simulink model "ALL_JP360_DBW_V6_5_1103"  (R2022a)
settings: Solver=FixedStepAuto  StartTime=0.0  StopTime=inf  FixedStep=0.01  RelTol=1e-3  EnableMultiTasking=on
model workspace (MAT data in the model file):
  g = 9.8
undefined symbols (not defined in the file or in its folder): canChannel, delta_v_p, IPM_Line_C0, IPM_Line_C1, IPM_Line_C2, IPM_Line_C3, M, M_p, MRR_ObjDistX, MRR_ObjDistY, MRR_ObjFusionCamID, MRR_ObjFusionSig, MRR_ObjID, MRR_ObjRelVelX, MRR_ObjRelVelY, MRR_ObjType, MRR_ObjUpdFlg, none, obj_vaild, untracktime, V, videoinput
libraries: canfdmsglib x230, canfdlib x76, slpidlib x24, simulink x18, dspstat3 x14, ctrlSharedLib x1, simulink_extras x1, imaqlib x1, realtime_pacer_lib x1, dspvision x1, visionsinks x1
(part 1 of 55)
settings Model: Creator=35528  LastModifiedBy=91388
settings SolverCC: PositivePriorityOrder=on  AutoInsertRateTranBlk=on
settings OptimizationCC: DefaultParameterBehavior=Inlined  GainParamInheritBuiltInType=on  UseFloatMulNetSlope=on  DefaultUnderspecifiedDataType=single  UseSpecifiedMinMax=on  InlineInvariantSignals=on  EnhancedBackFolding=on  CachingGlobalReferences=on  BitwiseOrLogicalOp=Bitwise operator  PassReuseOutputArgsAs=Individual arguments  ZeroExternalMemoryAtStartup=off  ZeroInternalMemoryAtStartup=off  NoFixptDivByZeroProtection=on  EfficientFloat2IntCast=on  OptimizeBlockOrder=speed  DifferentSizesBufferReuse=on  MultiThreadedLoops=on  EfficientTunableParamExpr=on
settings DebuggingCC: ParameterOverflowMsg=none  ParameterTunabilityLossMsg=error
settings ModelReferenceCC: ModelReferenceMinAlgLoopOccurrences=on
settings SFSimCC: MATLABDynamicMemAlloc=off
settings RTWCC: SystemTargetFile=ert.tlc  GenCodeOnly=on  PackageGeneratedCodeAndArtifacts=on  TemplateMakefile=ert_default_tmf  RetainRTWFile=on  BuildConfiguration=Faster Runs  CheckMdlBeforeBuild=Warning
settings CodeAppCC: ForceParamTrailComments=on  IgnoreCustomStorageClasses=off  OperatorAnnotations=on  SimulinkDataObjDesc=on  SFDataObjDesc=on  MATLABFcnDesc=on  InsertBlockDesc=on  StateflowObjectComments=on  MATLABSourceComments=on  ReqsInCode=on
settings ERTTargetCC: TargetLangStandard=C99 (ISO)  GenerateSampleERTMain=on  SuppressErrorStatus=on  SupportNonFinite=off  InlinedParameterPlacement=NonHierarchical  MultiInstanceErrorCode=Warning  RootIOFormat=Part of model data structure  ERTCustomFileTemplate=example_file_process.tlc

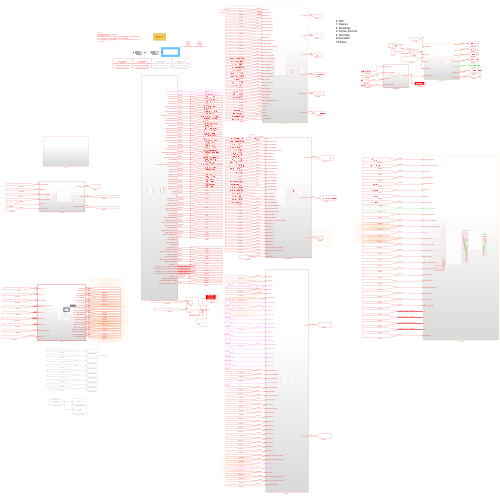
[thumbnail: Simulink's stored preview of the top-level diagram]
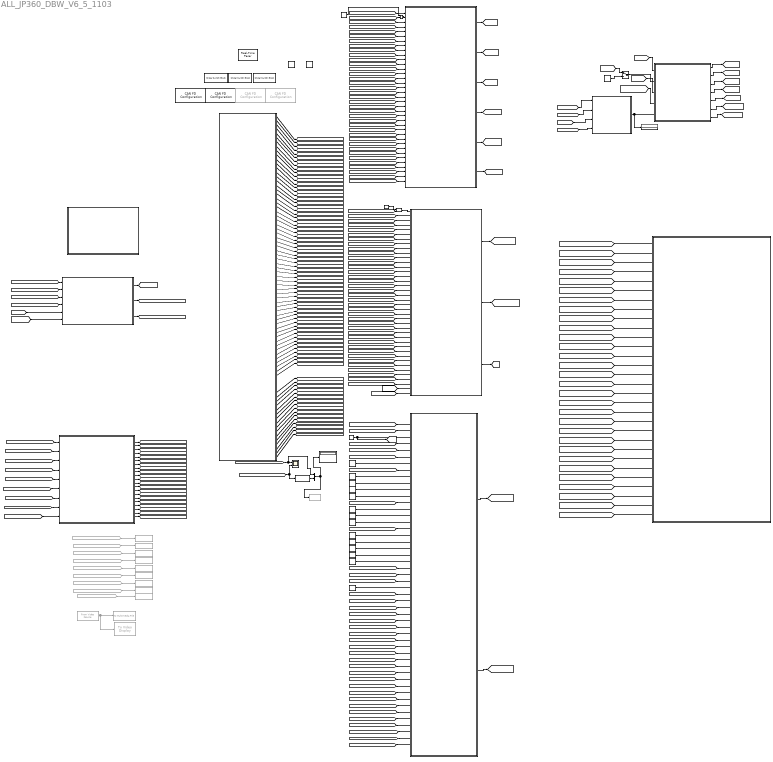
== system ALL_JP360_DBW_V6_5_1103 ==
  note: 0: OFF
      | 1: Passive
      | 2: Stand-By
      | 3: Active-Control
      | 5: Override
      | 6: Standstill
      | 7: Failure
  note: 注意事项
      | 1.添加Real-Time Pacer文件夹到路径下
      | 2.双击20230916.mat文件
      | 3.连接CANoe硬件（每次打开模型前最好电脑连接CANoe硬件，否则CAN配置会变），channel3对应公CAN，channel4对应1V1R私有CAN
      | 4.如果发现CAN配置变为了MathWork...，那么运行ALL_JP360_DBW_V2_2m.m文件，运行两次！！！！！！！！！
  ACC : Constant  OutDataTypeStr=boolean
  ACC_Control : Subsystem
  CAN FD Configuration1 : canfdlib/CAN FD Configuration  Device=Vector VN1640A 1 (Channel 3)  DeviceMenu=Vector VN1640A 1 (Channel 3)  BusFrequency=20  ObjConstructor=canChannel('Vector', 'VN1640A 1', 3, 'ProtocolMode', 'CAN FD')  ArbitrationBusSpeed=500000  ArbitrationPrescaler=5  ArbitrationSJW=8  ArbitrationTSEG1=31  ArbitrationTSEG2=8  DataBusSpeed=2000000  DataPrescaler=2  DataSJW=2  DataTSEG1=7  DataTSEG2=2  AckMode=Normal  BlockHandle=69358.0004
      settings: SourceProductBaseCode=VN
  CAN FD Configuration2 : canfdlib/CAN FD Configuration  Device=Vector VN1640A 1 (Channel 4)  DeviceMenu=Vector VN1640A 1 (Channel 4)  BusFrequency=20  ObjConstructor=canChannel('Vector', 'VN1640A 1', 4, 'ProtocolMode', 'CAN FD')  ArbitrationBusSpeed=500000  ArbitrationPrescaler=5  ArbitrationSJW=8  ArbitrationTSEG1=31  ArbitrationTSEG2=8  DataBusSpeed=2000000  DataPrescaler=2  DataSJW=2  DataTSEG1=7  DataTSEG2=2  AckMode=Normal  BlockHandle=69359.0004
      settings: SourceProductBaseCode=VN
  CAN FD Configuration3 : canfdlib/CAN FD Configuration  Commented=on  Device=MathWorks Virtual 1 (Channel 1)  DeviceMenu=MathWorks Virtual 1 (Channel 1)  BusFrequency=20  ObjConstructor=canChannel('MathWorks', 'Virtual 1', 1, 'ProtocolMode', 'CAN FD')  ArbitrationBusSpeed=1000000  ArbitrationPrescaler=5  ArbitrationSJW=8  ArbitrationTSEG1=31  ArbitrationTSEG2=8  DataBusSpeed=8000000  DataPrescaler=2  DataSJW=2  DataTSEG1=7  DataTSEG2=2  AckMode=Normal  BlockHandle=69360.0004
      settings: SourceProductBaseCode=VN
  CAN FD Configuration4 : canfdlib/CAN FD Configuration  Commented=on  Device=MathWorks Virtual 1 (Channel 1)  DeviceMenu=MathWorks Virtual 1 (Channel 1)  BusFrequency=20  ObjConstructor=canChannel('MathWorks', 'Virtual 1', 1, 'ProtocolMode', 'CAN FD')  ArbitrationBusSpeed=1000000  ArbitrationPrescaler=5  ArbitrationSJW=8  ArbitrationTSEG1=31  ArbitrationTSEG2=8  DataBusSpeed=8000000  DataPrescaler=2  DataSJW=2  DataTSEG1=7  DataTSEG2=2  AckMode=Normal  BlockHandle=69361.0004
      settings: SourceProductBaseCode=VN
  CIPV1 : Subsystem  TreatAsAtomicUnit=on
  CanbusControl : Subsystem
  Constant{10,44,47..48} (4 alike) : Constant  Value=150  OutDataTypeStr=single
  Constant{11,15,21,32} (4 alike) : Constant  Value=100  OutDataTypeStr=single
  Constant{12,19,22,33} (4 alike) : Constant  Value=20  OutDataTypeStr=single
  Constant40 : Constant  Value=0  OutDataTypeStr=int8
  Constant43 : Constant  Value=0  OutDataTypeStr=single
  Constant7 : Constant  OutDataTypeStr=single
  DCLC : Constant  OutDataTypeStr=boolean
  DCLC1 : Subsystem
  Data Store Memory : DataStoreMemory  DataStoreName=acc_change_mode  ReadBeforeWriteMsg=warning  WriteAfterWriteMsg=warning  WriteAfterReadMsg=warning  ShowAdditionalParam=off
  Data Store Memory1 : DataStoreMemory  DataStoreName=SpdSetValue  ReadBeforeWriteMsg=warning  WriteAfterWriteMsg=warning  WriteAfterReadMsg=warning  ShowAdditionalParam=off
  Data Type Conversion : DataTypeConversion  OutDataTypeStr=single  SaturateOnIntegerOverflow=off  RndMeth=Floor
  Display : Display
  Display1 : Display
  Error : Subsystem
  From Video Device : imaqlib/From Video Device  Commented=on  DeviceMenu=(none)  Device=winvideo 2 (SY 1080P camera)  ObjConstructor=videoinput('winvideo', 2)  VideoFormatMenu=(none)  VideoFormat=YUY2_352x288  VideoSource=input1  ROIPosition=[0 0 288 352]  EnableHWTrigger=off  TriggerConfiguration=none/none  SampleTime=0.03  OutputPortsMode=One multidimensional signal  DataType=single  CanDoHWTrigger=no  ReturnedColorSpace=rgb  BlockHandle=66699.0001  ROIWidth=352  ROIHeight=288  ROIColumn=0  ROIRow=0  EngXMLPath=D:\Program Files\MATLAB\R2022a\toolbox\imaq\imaq\private  DevXMLPath=C:\ProgramData\MATLAB\SupportPackages\R2022a\toolbox\imaq\supportpackages\genericvideo\adaptor\win64  EngLibPath=D:\Program Files\MATLAB\R2022a\toolbox\imaq\imaqblks\imaqmex\win64  ColorSpace=rgb  BayerSensorAlignment=grbg  ImaqMode=off
  From109 : From  Commented=on  GotoTag=MRR_obj_1_32
  From113 : From  Commented=on  GotoTag=ABS_VehSpdLgt
  From161 : From  Commented=on  GotoTag=ESP_YawRate
  From162 : From  Commented=on  GotoTag=VR_ADCU_IPM_Line_01_0x640FromOutData
  From163 : From  Commented=on  GotoTag=VR_ADCU_IPM_Line_02_0x641FromOutData
  From164 : From  Commented=on  GotoTag=VR_ADCU_IPM_Line_03_0x642FromOutData
  From165 : From  Commented=on  GotoTag=VR_ADCU_IPM_Line_04_0x643FromOutData
  From166 : From  Commented=on  GotoTag=SAS_SteerWheelAngle
  From167 : From  Commented=on  GotoTag=IPM_obj_1_20
  LKA : Constant  OutDataTypeStr=boolean
  LKA_Control : Subsystem
  Manual Switch : ManualSwitch
  MsgFromCAN : Subsystem
  MsgToCAN : Subsystem
  Mux : Mux  Inputs=2
  Product : Product
  Product1 : Product
  Real-Time Pacer : realtime_pacer_lib/Real-Time Pacer  simTimePerRealTime=1
      settings: SourceProductName=Real-Time Pacer
  Scope : Scope  NumInputPorts=2
  Slider Switch : SliderSwitchBlock
      settings: Values={{'Off', 'On'}, [0 1]}
  Slider Switch1 : SliderSwitchBlock
      settings: Values={{'Off', 'On'}, [0 1]}
  Slider Switch2 : SliderSwitchBlock
      settings: Values={{'Off', 'On'}, [0 1]}
  Subsystem1 : Subsystem
  To File : ToFile  Commented=on  Filename=EMS_HMI110_2.mat  SaveFormat=Timeseries
  To Multimedia File : dspvision/To Multimedia File  Commented=on  outputFilename=output.avi  streamSelection=Video only  videoCompressor=None (uncompressed)  audioCompressor=None (uncompressed)  imagePorts=One multidimensional signal  fileType=AVI  audioDatatype=16-bit integer  fourcc=RGB  videoQuality=75  mj2000CompFactor=10
  To Video Display : visionsinks/To Video Display  Commented=on  windowSizeMode=Normal  openAtMdlStart=on  fullScreen=off  videoWindowX=536805376  videoWindowY=536805376  saveWindowSize=off  videoWindowWidth=1280  videoWindowHeight=720  inputColorFormat=RGB  inputType=Obsolete  imagePorts=One multidimensional signal  OutputDevice=On-screen video monitor  dataOrg=Column-major  isWindowOpen=off
  To Workspace1 : ToWorkspace  Commented=on  VariableName=MRR_obj_1_32  SaveFormat=Timeseries  SampleTime=-1
  To Workspace2 : ToWorkspace  Commented=on  VariableName=ABS_VehSpdLgt  SaveFormat=Timeseries  SampleTime=-1
  To Workspace3 : ToWorkspace  Commented=on  VariableName=ESP_YawRate  SaveFormat=Timeseries  SampleTime=-1
  To Workspace4 : ToWorkspace  Commented=on  VariableName=VR_ADCU_IPM_Line_01_0x640FromOutData  SaveFormat=Timeseries  SampleTime=-1
  To Workspace5 : ToWorkspace  Commented=on  VariableName=VR_ADCU_IPM_Line_02_0x641FromOutData  SaveFormat=Timeseries  SampleTime=-1
  To Workspace6 : ToWorkspace  Commented=on  VariableName=VR_ADCU_IPM_Line_03_0x642FromOutData  SaveFormat=Timeseries  SampleTime=-1
  To Workspace7 : ToWorkspace  Commented=on  VariableName=VR_ADCU_IPM_Line_04_0x643FromOutData  SaveFormat=Timeseries  SampleTime=-1
  To Workspace8 : ToWorkspace  Commented=on  VariableName=SAS_SteerWheelAngle  SaveFormat=Timeseries  SampleTime=-1
  To Workspace9 : ToWorkspace  Commented=on  VariableName=IPM_obj_1_20  SaveFormat=Timeseries  SampleTime=-1
  button : Subsystem
  wires:
  [IPM_obj_1_20] -> CIPV1/9(IPM_obj_1_20)
  MsgFromCAN/43(Output8) -> [ESP_Algt]
  [EMS_IndicatedEngError] -> ACC_Control/16(EMS_IndicatedEngError)
  [CIPV_ObjRelVelX] -> ACC_Control/30(CIPV_velocity)
  MsgFromCAN/74(VR_ADCU_IPM_Line_02_0x641FromOutData) -> [VR_ADCU_IPM_Line_02_0x641FromOutData]
  CanbusControl/1(Lanelist_Out) -> [Lanelist_Out]
  [VR_ADCU_IPM_Line_01_0x640FromOutData] -> CIPV1/4(IPM_Line_01)
  [ESP_YawRate] -> CIPV1/3(ESP_YawRate)
  [BCM_DoorStsRearRi] -> ACC_Control/8(BCM_DoorStsRearRi)
  CIPV1/10(Left_closest_ObjDistY) -> [Left_closest_ObjDistY]
  [ESP_Algt] -> ACC_Control/34(ay_esp)
  ACC_Control/6(ACC_DriveOff) -> [ACC_DriveOff]
  MsgFromCAN/11(Output7) -> [ESP_Master_Cylinder_Pressure]
  [SWM_ACCResume] -> ACC_Control/4(SWM_ACCResume)
  CanbusControl/7(Torque_Status) -> [Torque_Status]
  MsgFromCAN/7(Output1) -> [BCM_TurnIndicatorSts]
  MsgFromCAN/5(Out6) -> [IPM_Line04_C0]
  CIPV1/11(Left_closest_ObjRelVelX) -> [Left_closest_ObjRelVelX]
  MsgFromCAN/79(Out15) -> [IPM_Line03_Existence_Probability]
  [ESP_EPBStatus] -> ACC_Control/21(ESP_EPBStatus)
  CIPV1/13(ACC_left_ObjDetected) -> [ACC_left_ObjDetected]
  [ESP_EspEnableSts] -> ACC_Control/22(ESP_EspEnableSts)
  MsgFromCAN/80(Out16) -> [IPM_Line04_Existence_Probability]
  [ACC_ObjDetected1] -> ACC_Control/28(CIPV_detected_flag)
  [CIPV_ObjDistX] -> ACC_Control/29(CIPV_distance)
  MsgFromCAN/66(Out21) -> [IPM_Line01_ColorClass]
  [SWM_ACCvSetMinus] -> button/4(SWM_ACCvSetMinus)
  [acc_status] -> CanbusControl/1(ACCstatus_in)
  ACC/1 -> Product/1
  MsgFromCAN/56(Output25) -> [BCM_PowerModeInvalid]
  [SWM_ACCtauGapSetMinus] -> button/2(TimeGapSet)
  CIPV1/16(Right_closest_ObjDistX) -> [Right_closest_ObjDistX]
  From166/1 -> To Workspace8/1
  [VR_ADCU_IPM_Line_03_0x642FromOutData] -> CIPV1/6(PM_Line_03)
  [VR_ADCU_IPM_Line_02_0x641FromOutData] -> CIPV1/5(IPM_Line_02)
  MsgFromCAN/6(Out7) -> [IPM_Line04_C1]
  CIPV1/9(Left_closest_ObjDistX) -> [Left_closest_ObjDistX]
  From162/1 -> To Workspace4/1
  [BCM_PowerMode] -> ACC_Control/12(BCM_PowerMode)
  MsgFromCAN/22(Output20) -> [ESP_YawRate]
  Product/1 -> ACC_Control/2(SWM_ACCSwitch)
  CanbusControl/5(ACC_StartStop) -> [ACC_StartStop]
  button/2(setvspeed) -> [setvspeed]
  CanbusControl/4(Brake_Status) -> [Brake_Status]
  From161/1 -> To Workspace3/1
  From109/1 -> To Workspace1/1
  CIPV1/3(CIPV_ObjDistY) -> [CIPV_ObjDistY]
  [EMS_BrkPedalStasus] -> ACC_Control/18(EMS_BrkPedalStasus)
  MsgFromCAN/24(Output22) -> [ABS_AbsCtrlActv]
  From163/1 -> To Workspace5/1
  MsgFromCAN/40(Out13) -> [IPM_Line02_C2]
  CIPV1/1(CIPV_ObjID) -> [CIPV_ObjID]
  [IC_VehSpd_HMI] -> ACC_Control/37(IC_VehSpd_HMI)
  CIPV1/2(CIPV_ObjDistX) -> [CIPV_ObjDistX]
  [IC_VehSpd_HMI] -> Scope/2, Data Type Conversion/1
  [IPM_LineAssit_Status] -> CanbusControl/4(LKAstatus_in)
  [BCM_PowerModeInvalid] -> ACC_Control/11(BCM_PowerModeInvalid)
  [ABS_VehSpdLgt] -> CIPV1/2(Ego_speed)
  Data Type Conversion/1 -> Mux/2
  [EMS_IndicatedDriverOverride] -> ACC_Control/31(EMS_IndicatedDriverOverride)
  MsgFromCAN/78(Output33) -> [EMS_IndicatedRealEngTorq]
  Constant7/1 -> Manual Switch/2
  [acc_torque] -> Manual Switch/1
  CIPV1/7(CIPV_ObjType) -> [CIPV_ObjType]
  CIPV1/12(Left_closest_ObjRelVelY) -> [Left_closest_ObjRelVelY]
  CIPV1/19(Right_closest_ObjRelVelY) -> [Right_closest_ObjRelVelY]
  CIPV1/15(Right_closest_ObjID) -> [Right_closest_ObjID]
  CIPV1/17(Right_closest_ObjDistY) -> [Right_closest_ObjDistY]
  CanbusControl/2(Torque_Out) -> [Torque_Out]
  From165/1 -> To Workspace7/1
  CIPV1/5(CIPV_ObjRelVelY) -> [CIPV_ObjRelVelY]
  [ESP_Alat] -> ACC_Control/33(ax_esp)
  CIPV1/21(Right_closest_ObjType) -> [Right_closest_ObjType]
  [set_speed_out] -> button/6(set_speed_out)
  [ABS_VehSpdDirection] -> ACC_Control/23(ABS_VehSpdDirection)
  CIPV1/4(CIPV_ObjRelVelX) -> [CIPV_ObjRelVelX]
  [MRR_obj_1_32] -> CIPV1/1(MRR_obj_1_32)
  MsgFromCAN/75(VR_ADCU_IPM_Line_03_0x642FromOutData) -> [VR_ADCU_IPM_Line_03_0x642FromOutData]
  MsgFromCAN/77(IPM_obj_1_20) -> [IPM_obj_1_20]
  [ESP_AvhActive] -> ACC_Control/24(ESP_AvhActive)
  [BCM_DoorStsRearLe] -> ACC_Control/7(BCM_DoorStsRearLe)
  [setvspeed] -> ACC_Control/32(set_speed_in)
  From Video Device/1 -> To Video Display/1, To Multimedia File/1
  [SWM_ACCSet] -> ACC_Control/3(SWM_ACCSet)
  [SWM_ACCSwitchOut] -> Product/2
  CIPV1/8(Left_closest_ObjID) -> [Left_closest_ObjID]
  From164/1 -> To Workspace6/1
  MsgFromCAN/8(ESP_YawRateStatus) -> [ESP_YawRateStatus]
  MsgFromCAN/53(Output21) -> [EMS_AccRAWPedalRatio]
  MsgFromCAN/72(MRR_obj_1_32) -> [MRR_obj_1_32]
  [SAS_SteerWheelAngle] -> CIPV1/8(SAS_SteerWheelAngle)
  MsgFromCAN/35(Out8) -> [IPM_Line01_C1]
  MsgFromCAN/70(Out25) -> [IPM_Line02_Existence_Probability]
  MsgFromCAN/67(Out22) -> [IPM_Line01_Existence_Probability]
  [acc_status] -> button/5(acc_status)
  [TimeGapSet] -> ACC_Control/26(HWT_dem[s])
  MsgFromCAN/71(Output32) -> [SWM_TurnIndicationAct]
  [BCM_EnginehoodSts] -> ACC_Control/14(BCM_EnginehoodSts)
  MsgFromCAN/69(Out24) -> [IPM_Line02_ColorClass]
  From113/1 -> To Workspace2/1
  MsgFromCAN/61(EMS_IndicatedEngError1) -> [IC_VehSpd_HMI]
  MsgFromCAN/17(Output15) -> [BCM_DoorStsFrntLe]
  button/3(Out3) -> [SWM_ACCSwitchOut]
  MsgFromCAN/3(Out4) -> [IPM_Line03_C0]
  CanbusControl/6(Lanelist_Status) -> [Lanelist_Status]
  MsgFromCAN/27(EPS_LKAControlStatus) -> [EPS_LKAControlStatus]
  Mux/1 -> To File/1, Display/1
  [setvspeed] -> ACC_Control/27(Des_speed[m/s])
  [SWM_ACCvSetPlus] -> button/3(SWM_ACCvSetPlus)
  [EMS_IndicatedRealEngTorq] -> Mux/1, Scope/1
  Manual Switch/1 -> CanbusControl/2(Torque_in)
  button/1(TimeGapSetOut) -> [TimeGapSet]
  CIPV1/14(Left_closest_ObjType) -> [Left_closest_ObjType]
  [EPS_EPSPAMSts] -> ACC_Control/19(EPS_EPSPAMSts)
  ACC_Control/2(acc_torque) -> [acc_torque]
  [TCU_GearSelectorReq] -> ACC_Control/20(TCU_GearSelectorReq)
  [SRS_SBR_Driver] -> ACC_Control/15(SRS_SBR_Driver)
  ACC_Control/4(set_speed_out) -> [set_speed_out]
  ACC_Control/3(acc_brake) -> [acc_brake]
  MsgFromCAN/60(Output29) -> [SWM_ACCtauGapSetMinus]
  ACC_Control/1(acc_status) -> [acc_status]
  MsgFromCAN/12(TCU_GearSelectorReq) -> [TCU_GearSelectorReq]
  MsgFromCAN/52(ESP_EspCtrlActv2) -> [ESP_AvhActive]
  [VR_ADCU_IPM_Line_04_0x643FromOutData] -> CIPV1/7(IPM_Line_04)
  MsgFromCAN/44(Output) -> [SWM_LaneAssistSwitch]
  [MRR_HWFail] -> ACC_Control/10(MRR_HWFail)
  [BCM_DoorStsFrntLe] -> ACC_Control/5(BCM_DoorStsFrntLe)
  [EMS_AccRAWPedalRatio] -> ACC_Control/17(EMS_AccRAWPedalRatio)
  MsgFromCAN/54(Output23) -> [EMS_BrkPedalStasus]
  MsgFromCAN/73(VR_ADCU_IPM_Line_01_0x640FromOutData) -> [VR_ADCU_IPM_Line_01_0x640FromOutData]
  [BCM_Mechanical_Hand_Brake] -> ACC_Control/13(BCM_Mechanical_Hand_Brake)
  From167/1 -> To Workspace9/1
  MsgFromCAN/33(Output5) -> [MRR_HWFail]
  MsgFromCAN/58(Output27) -> [BCM_Mechanical_Hand_Brake]
  [ESP_YawRate] -> ACC_Control/35(yaw_rate)
  MsgFromCAN/34(Out1) -> [IPM_Line01_C0]
  CIPV1/18(Right_closest_ObjRelVelX) -> [Right_closest_ObjRelVelX]
  MsgFromCAN/41(Out14) -> [IPM_Line02_C3]
  MsgFromCAN/37(Out10) -> [IPM_Line01_C3]
  CanbusControl/3(Brake_Out) -> [Brake_Out]
  MsgFromCAN/55(Output24) -> [EMS_IndicatedDriverOverride]
  MsgFromCAN/38(Out11) -> [IPM_Line02_C0]
  MsgFromCAN/4(Out5) -> [IPM_Line03_C1]
  MsgFromCAN/59(Output28) -> [ABS_VehSpdDirection]
  MsgFromCAN/57(Output26) -> [BCM_PowerMode]
  [ESP_VehicleStandstill] -> ACC_Control/25(ESP_VehicleStandstill)
  MsgFromCAN/13(SAS_SteerWheelRotSpd) -> [SAS_SteerWheelRotSpd]
  MsgFromCAN/9(Output3) -> [ABS_VehSpdLgtStatus]
  MsgFromCAN/21(Output19) -> [BCM_EnginehoodSts]
  MsgFromCAN/28(EPS_LKAResponseTorque) -> [EPS_LKAResponseTorque]
  MsgFromCAN/50(Output14) -> [ESP_VehicleStandstill]
  MsgFromCAN/48(Output12) -> [SWM_ACCvSetPlus]
  MsgFromCAN/30(ESP_EspEnableSts) -> [ESP_EspEnableSts]
  MsgFromCAN/76(VR_ADCU_IPM_Line_04_0x643FromOutData) -> [VR_ADCU_IPM_Line_04_0x643FromOutData]
  MsgFromCAN/16(EMS_IndicatedEngError) -> [EMS_IndicatedEngError]
  MsgFromCAN/29(EPS_EPSPAMSts) -> [EPS_EPSPAMSts]
  MsgFromCAN/2(Out3) -> [RRR_SystemStatus]
  MsgFromCAN/51(ESP_EspCtrlActv1) -> [ESP_EPBStatus]
  [SAS_SteerWheelAngle] -> ACC_Control/36(steer_angle)
  MsgFromCAN/25(SAS_SteerWheelAngle) -> [SAS_SteerWheelAngle]
  MsgFromCAN/68(Out23) -> [IPM_Line02_Type]
  MsgFromCAN/20(Output18) -> [BCM_DoorStsRearLe]
  MsgFromCAN/49(Output13) -> [SWM_ACCvSetMinus]
  ACC_Control/5(standstill_req) -> [standstill_req]
  MsgFromCAN/39(Out12) -> [IPM_Line02_C1]
  MsgFromCAN/42(Output2) -> [ESP_Alat]
  [BCM_DoorStsFrntRi] -> ACC_Control/6(BCM_DoorStsFrntRi)
  [acc_brake] -> CanbusControl/3(Brake_in)
  MsgFromCAN/15(ESP_EspCtrlActv) -> [ESP_EspCtrlActv]
  MsgFromCAN/31(ESP_Master_Cylinder_Pressure_Status) -> [ESP_Master_Cylinder_Pressure_Status]
  MsgFromCAN/26(Output4) -> [SAS_SteerWheelRotSpdStatus]
  MsgFromCAN/45(Output9) -> [SWM_ACCResume]
  MsgFromCAN/23(ABS_VehSpdLgt) -> [ABS_VehSpdLgt]
  MsgFromCAN/36(Out9) -> [IPM_Line01_C2]
  MsgFromCAN/10(SRS_SBR_Driver) -> [SRS_SBR_Driver]
  CIPV1/6(ACC_ObjDetected) -> [ACC_ObjDetected1]
  MsgFromCAN/19(Output17) -> [BCM_DoorStsFrntRi]
  MsgFromCAN/18(Output16) -> [BCM_DoorStsRearRi]
  MsgFromCAN/14(EPS_TorsionBarTorque) -> [EPS_TorsionBarTorque]
  [SWM_ACCSwitch] -> button/1(SWM_ACCSwitch)
  CIPV1/20(ACC_right_ObjDetected) -> [ACC_right_ObjDetected]
  MsgFromCAN/32(Output6) -> [IPM_SensorState]
  MsgFromCAN/46(Output10) -> [SWM_ACCSet]
  MsgFromCAN/1(Out2) -> [FRR_SystemStatus]
  MsgFromCAN/65(Out20) -> [IPM_Line01_Type]
  [IPM_SensorState] -> ACC_Control/9(IPM_SensorState)
  MsgFromCAN/47(Output11) -> [SWM_ACCSwitch]
  [ABS_VehSpdLgt] -> ACC_Control/1(Ego_speed)
  [standstill_req] -> MsgToCAN/5(ACC_StandstillReq)
  [ACC_ObjDetected1] -> MsgToCAN/14(ACC_ObjDetected)
  [Brake_Out] -> MsgToCAN/3(ACC_TgtAx)
  [VR_ADCU_IPM_Line_04_0x643FromOutData] -> MsgToCAN/29(643)
  [Right_closest_ObjType] -> MsgToCAN/19(MRR_R_Obj_0x_class)
  [ACC_StartStop] -> MsgToCAN/9(ACC_EngineStartstop)
  [CIPV_ObjDistX] -> MsgToCAN/23(MRR_F_Object_dx)
  [Torque_Out] -> MsgToCAN/1(ACC_Torque_Request)
  [Left_closest_ObjType] -> MsgToCAN/15(MRR_L_Obj_0x_class)
  [Right_closest_ObjDistY] -> MsgToCAN/21(MRR_R_Object_dy)
  [VR_ADCU_IPM_Line_03_0x642FromOutData] -> MsgToCAN/28(642)
  [CIPV_ObjDistY] -> MsgToCAN/24(MRR_F_Object_dy)
  [VR_ADCU_IPM_Line_02_0x641FromOutData] -> MsgToCAN/27(641)
  [Torque_Status] -> MsgToCAN/2(ACC_Torque_Request_Status)
  [ACC_left_ObjDetected] -> MsgToCAN/18(MRR_LeftTargetDetection)
  [ACC_DriveOff] -> MsgToCAN/30(ACC_DriveOff)
  [VR_ADCU_IPM_Line_01_0x640FromOutData] -> MsgToCAN/26(640)
  [Right_closest_ObjDistX] -> MsgToCAN/20(MRR_R_Object_dx)
  [ACC_right_ObjDetected] -> MsgToCAN/22(MRR_RightTargetDetection)
  [acc_status] -> MsgToCAN/6(ACC_Status)
  [TimeGapSet] -> MsgToCAN/8(ACC_TimeGapSet)
  [Left_closest_ObjDistX] -> MsgToCAN/16(MRR_L_Object_dx)
  [set_speed_out] -> MsgToCAN/7(setvspped)
  [Lanelist_Status] -> MsgToCAN/12(IPM_LaneAssit_TorqueReqStatus)
  [Obj_Speed] -> MsgToCAN/13(Obj_Speed)
  [IPM_LineAssit_Status] -> MsgToCAN/10(IPM_LaneAssit_Status)
  [Lanelist_Out] -> MsgToCAN/11(IPM_LaneAssit_TorqueReq)
  [Left_closest_ObjDistY] -> MsgToCAN/17(MRR_L_Object_dy)
  [CIPV_ObjType] -> MsgToCAN/25(MRR_F_Obj_0x_class)
  [Brake_Status] -> MsgToCAN/4(ACC_BrakePreferred)
  [IPM_SensorState] -> LKA_Control/8(IPM_SensorState)
  [BCM_DoorStsFrntRi] -> LKA_Control/16(BCM_DoorStsFrntRi)
  [ABS_VehSpdLgtStatus] -> LKA_Control/4(ABS_VehSpdLgtStatus)
  [EMS_IndicatedEngError] -> LKA_Control/13(EMS_IndicatedEngError)
  LKA_Control/1(LKAReq_angle) -> [LKAReq_angle]
  [ESP_EspEnableSts] -> LKA_Control/27(ESP_EspEnableSts)
  [SRS_SBR_Driver] -> LKA_Control/6(SRS_SBR_Driver)
  [BCM_DoorStsRearLe] -> LKA_Control/17(BCM_DoorStsRearLe)
  [ESP_YawRateStatus] -> LKA_Control/3(ESP_YawRateStatus)
  [ESP_Master_Cylinder_Pressure_Status] -> LKA_Control/28(ESP_Master_Cylinder_Pressure_Status)
  [EPS_LKAControlStatus] -> LKA_Control/24(EPS_LKAControlStatus)
  [ESP_YawRate] -> LKA_Control/19(ESP_YawRate)
  [BCM_DoorStsRearRi] -> LKA_Control/15(BCM_DoorStsRearRi)
  [SWM_TurnIndicationAct] -> LKA_Control/2(SWM_TurnIndicatorAct)
  [BCM_EnginehoodSts] -> LKA_Control/18(BCM_EnginehoodSts)
  [ESP_EspCtrlActv] -> LKA_Control/12(ESP_EspCtrlActv)
  [IPM_Line01_C3] -> LKA_Control/32(IPM_Line01_C3)
  [SAS_SteerWheelRotSpdStatus] -> LKA_Control/23(SAS_SteerWheelRotSpdStatus)
  [SWM_LaneAssistSwitch] -> Product1/2
  Product1/1 -> LKA_Control/1(SWM)
  [MRR_HWFail] -> LKA_Control/7(MRR_HWFail)
  [EPS_TorsionBarTorque] -> LKA_Control/11(EPS_TorsionBarTorque)
  [ESP_Master_Cylinder_Pressure] -> LKA_Control/5(ESP_Master_Cylinder_Pressure)
  [SAS_SteerWheelRotSpd] -> LKA_Control/10(SAS_SteerWheelRotSpd)
  [DCLC_status] -> LKA_Control/40(DCLC_Status)
  [IPM_Line01_C0] -> LKA_Control/29(IPM_Line01_C0)
  [IPM_Line02_C0] -> LKA_Control/33(IPM_Line02_C0)
  [SAS_SteerWheelAngle] -> LKA_Control/22(SAS_SteerWheelAngle)
  [IPM_Line02_Existence_Probability] -> LKA_Control/38(IPM_Line02_Existence_Probability)
  [TCU_GearSelectorReq] -> LKA_Control/9(TCU_GearSelectorReq)
  [EPS_EPSPAMSts] -> LKA_Control/26(EPS_EPSPAMSts)
  [IPM_Line01_Existence_Probability] -> LKA_Control/37(IPM_Line01_Existence_Probability)
  LKA_Control/3(err_now) -> [errnow]
  [EPS_LKAResponseTorque] -> LKA_Control/25(EPS_LKAResponseTorque)
  [IPM_Line02_C3] -> LKA_Control/36(IPM_Line02_C3)
  [acc_status] -> LKA_Control/39(acc_sta)
  [ABS_AbsCtrlActv] -> LKA_Control/21(ABS_AbsCtrlActv)
  [BCM_DoorStsFrntLe] -> LKA_Control/14(BCM_DoorStsFrntLe)
  LKA_Control/2(IPM_LineAssit_Status) -> [IPM_LineAssit_Status]
  [IPM_Line02_C1] -> LKA_Control/34(IPM_Line02_C1)
  [IPM_Line01_C1] -> LKA_Control/30(IPM_Line01_C1)
  [IPM_Line01_C2] -> LKA_Control/31(IPM_Line01_C2)
  LKA/1 -> Product1/1
  [ABS_VehSpdLgt] -> LKA_Control/20(ABS_VehSpdLgt)
  [IPM_Line02_C2] -> LKA_Control/35(IPM_Line02_C2)
  [DCLC_status] -> Subsystem1/3(DCLC_status)
  [DCLCRequestTorque] -> Subsystem1/4(DCLCRequestTorque)
  [IPM_LineAssit_Status] -> Subsystem1/2(IPM_LineAssit_Status)
  [LKAReq_angle] -> Subsystem1/1(LKAReq_angle)
  Subsystem1/1(torque_req) -> CanbusControl/5(LanelistTorque_in), Display1/1
  [IPM_Line02_ColorClass] -> DCLC1/32(IPM_Line02_ColorClass)
  Constant19/1 -> DCLC1/19(RRR_OBJ1_Dy)
  [IPM_Line02_C0] -> DCLC1/36(IPM_Line02_C0)
  [MRR_HWFail] -> DCLC1/47(MRR_HWFail)
  [ESP_Alat] -> DCLC1/5(ESP_Alat)
  [IPM_Line04_C1] -> DCLC1/42(IPM_Line04_C1)
  [IPM_Line03_C1] -> DCLC1/41(IPM_Line03_C1)
  [IPM_Line01_Existence_Probability] -> DCLC1/43(IPM_Line01_Existence_Probability)
  DCLC1/1(torque) -> [DCLCRequestTorque]
  Constant11/1 -> DCLC1/21(RLR_OBJ1_Dx)
  [ABS_VehSpdLgt] -> DCLC1/6(ABS_VehSpdLgt)
  Constant44/1 -> DCLC1/9(FLR_ObjRelVel)
  [IPM_SensorState] -> DCLC1/28(IPM_SensorState)
  [FRR_SystemStatus] -> DCLC1/13(FRR_SystemStatus)
  [EMS_AccRAWPedalRatio] -> DCLC1/24(EMS_AccRAWPedalRatio)
  [EMS_BrkPedalStasus] -> DCLC1/23(EMS_BrkPedalStasus)
  [SAS_SteerWheelAngle] -> DCLC1/50(SAS_SteerWheelAngle1)
  DCLC1/2(DCLC_status) -> [DCLC_status]
  Constant47/1 -> DCLC1/12(FRR_ObjRelVel)
  [IPM_LineAssit_Status] -> DCLC1/2(LKA_Enable)
  [EPS_TorsionBarTorque] -> DCLC1/27(EPS_TorsionBarTorque)
  [IPM_Line01_C2] -> DCLC1/31(IPM_Line01_C2)
  [ESP_Algt] -> DCLC1/4(ESP_Algt)
  [IPM_Line01_ColorClass] -> DCLC1/29(IPM_Line01_ColorClass)
  [IPM_Line01_C1] -> DCLC1/39(IPM_Line01_C1)
  [IPM_Line03_C0] -> DCLC1/37(IPM_Line03_C0)
  Constant22/1 -> DCLC1/15(FRR_OBJ1_Dy)
  [Obj_Speed] -> DCLC1/8(Obj_Speed)
  [IPM_Line01_Type] -> DCLC1/30(IPM_Line01_Type)
  Constant10/1 -> DCLC1/20(RLR_ObjRelVel)
  Constant48/1 -> DCLC1/16(RRR_ObjRelVel)
  [MRR_F_Object_dy] -> DCLC1/46(MRR_F_Object_dy)
  Constant40/1 -> DCLC1/26(BCM_TurnIndicatorDig)
  Constant33/1 -> DCLC1/11(FLR_OBJ1_Dy)
  [IPM_Line01_C0] -> DCLC1/35(IPM_Line01_C0)
  Constant15/1 -> DCLC1/18(RRR_OBJ1_Dx)
  [acc_status] -> DCLC1/1(ACC_Enable)
  [MRR_F_Object_dx] -> DCLC1/45(MRR_F_Object_dx)
  Constant21/1 -> DCLC1/14(FRR_OBJ1_Dx)
  [IPM_Line04_Existence_Probability] -> DCLC1/49(IPM_Line04_Existence_Probability)
  [IPM_Line03_Existence_Probability] -> DCLC1/48(IPM_Line03_Existence_Probability)
  [IPM_Line02_C2] -> DCLC1/34(IPM_Line02_C2)
  [IPM_Line02_Existence_Probability] -> DCLC1/44(IPM_Line02_Existence_Probability)
  [IPM_Line02_Type] -> DCLC1/33(IPM_Line02_Type)
  Constant32/1 -> DCLC1/10(FLR_OBJ1_Dx)
  [IPM_Line02_C1] -> DCLC1/40(IPM_Line02_C1)
  DCLC/1 -> DCLC1/3(DCLC_Enable), [DCLC]
  [SWM_TurnIndicationAct] -> DCLC1/25(BCM_TurnIndicatorSts)
  Constant43/1 -> DCLC1/7(ABS_VehSpdLat)
  [RRR_SystemStatus] -> DCLC1/17(RRR_SystemStatus)
  Constant12/1 -> DCLC1/22(RLR_OBJ1_Dy)
  [IPM_Line04_C0] -> DCLC1/38(IPM_Line04_C0)

== system ALL_JP360_DBW_V6_5_1103/ACC_Control ==
  Ego_speed : Inport
  SWM_ACCSwitch : Inport  Port=2
  SWM_ACCSet : Inport  Port=3
  SWM_ACCResume : Inport  Port=4
  BCM_DoorStsFrntLe : Inport  Port=5
  BCM_DoorStsFrntRi : Inport  Port=6
  BCM_DoorStsRearLe : Inport  Port=7
  BCM_DoorStsRearRi : Inport  Port=8
  IPM_SensorState : Inport  Port=9
  MRR_HWFail : Inport  Port=10
  BCM_PowerModeInvalid : Inport  Port=11
  BCM_PowerMode : Inport  Port=12
  BCM_Mechanical_Hand_Brake : Inport  Port=13
  BCM_EnginehoodSts : Inport  Port=14
  SRS_SBR_Driver : Inport  Port=15
  EMS_IndicatedEngError : Inport  Port=16
  EMS_AccRAWPedalRatio : Inport  Port=17
  EMS_BrkPedalStasus : Inport  Port=18
  EPS_EPSPAMSts : Inport  Port=19
  TCU_GearSelectorReq : Inport  Port=20
  ESP_EPBStatus : Inport  Port=21
  ESP_EspEnableSts : Inport  Port=22
  ABS_VehSpdDirection : Inport  Port=23
  ESP_AvhActive : Inport  Port=24
  ESP_VehicleStandstill : Inport  Port=25
  HWT_dem[s] : Inport  Port=26
  Des_speed[m/s] : Inport  Port=27
  CIPV_detected_flag : Inport  Port=28
  CIPV_distance : Inport  Port=29
  CIPV_velocity : Inport  Port=30
  EMS_IndicatedDriverOverride : Inport  Port=31
  set_speed_in : Inport  Port=32
  ax_esp : Inport  Port=33
  ay_esp : Inport  Port=34
  yaw_rate : Inport  Port=35
  steer_angle : Inport  Port=36
  IC_VehSpd_HMI : Inport  Port=37
  ACC_FUNCTION : Subsystem
  Scope{,1..5} (6 alike) : Scope
  Scope6 : Scope  NumInputPorts=5
  acc_status : Outport
  acc_torque : Outport  Port=2
  acc_brake : Outport  Port=3
  set_speed_out : Outport  Port=4
  standstill_req : Outport  Port=5
  ACC_DriveOff : Outport  Port=6
  wires:
  BCM_PowerMode/1 -> ACC_FUNCTION/12(BCM_PowerMode)
  BCM_EnginehoodSts/1 -> ACC_FUNCTION/14(BCM_EnginehoodSts)
  CIPV_distance/1 -> ACC_FUNCTION/29(CIPV_distance)
  ESP_AvhActive/1 -> ACC_FUNCTION/24(ESP_AvhActive)
  Des_speed[m/s]/1 -> ACC_FUNCTION/27(Des_speed[km/h])
  EMS_AccRAWPedalRatio/1 -> ACC_FUNCTION/17(EMS_AccRAWPedalRatio)
  BCM_DoorStsFrntLe/1 -> ACC_FUNCTION/5(BCM_DoorStsFrntLe)
  BCM_Mechanical_Hand_Brake/1 -> ACC_FUNCTION/13(BCM_Mechanical_Hand_Brake)
  CIPV_velocity/1 -> Scope/1, ACC_FUNCTION/30(CIPV_velocity)
  set_speed_in/1 -> ACC_FUNCTION/32(set_speed_in)
  BCM_DoorStsFrntRi/1 -> ACC_FUNCTION/6(BCM_DoorStsFrntRi)
  SRS_SBR_Driver/1 -> ACC_FUNCTION/15(SRS_SBR_Driver)
  BCM_PowerModeInvalid/1 -> ACC_FUNCTION/11(BCM_PowerModeInvalid)
  BCM_DoorStsRearRi/1 -> ACC_FUNCTION/8(BCM_DoorStsRearRi)
  ESP_VehicleStandstill/1 -> Scope6/4, ACC_FUNCTION/25(ESP_VehicleStandstill), Scope5/1  "veh_standstill"
  ABS_VehSpdDirection/1 -> ACC_FUNCTION/23(ABS_VehSpdDirection)
  EMS_BrkPedalStasus/1 -> ACC_FUNCTION/18(EMS_BrkPedalStasus)
  EMS_IndicatedDriverOverride/1 -> ACC_FUNCTION/31(EMS_IndicatedDriverOverride)
  SWM_ACCResume/1 -> ACC_FUNCTION/4(SWM_ACCResume)
  EMS_IndicatedEngError/1 -> ACC_FUNCTION/16(EMS_IndicatedEngError)
  CIPV_detected_flag/1 -> ACC_FUNCTION/28(CIPV_detected_flag)
  BCM_DoorStsRearLe/1 -> ACC_FUNCTION/7(BCM_DoorStsRearLe)
  TCU_GearSelectorReq/1 -> ACC_FUNCTION/20(TCU_GearSelectorReq)
  ESP_EPBStatus/1 -> ACC_FUNCTION/21(ESP_EPBStatus)
  EPS_EPSPAMSts/1 -> ACC_FUNCTION/19(EPS_EPSPAMSts)
  SWM_ACCSet/1 -> ACC_FUNCTION/3(SWM_ACCSet)
  HWT_dem[s]/1 -> ACC_FUNCTION/26(HWT_dem[s])
  ESP_EspEnableSts/1 -> ACC_FUNCTION/22(ESP_EspEnableSts)
  MRR_HWFail/1 -> ACC_FUNCTION/10(MRR_HWFail)
  SWM_ACCSwitch/1 -> ACC_FUNCTION/2(SWM_ACCSwitch)
  IPM_SensorState/1 -> ACC_FUNCTION/9(IPM_SensorState)
  Ego_speed/1 -> ACC_FUNCTION/1(Ego_speed)
  ax_esp/1 -> ACC_FUNCTION/33(ax_esp)
  ay_esp/1 -> ACC_FUNCTION/34(ay_esp)
  yaw_rate/1 -> ACC_FUNCTION/35(yaw_rate)
  steer_angle/1 -> ACC_FUNCTION/36(steer_angle)
  ACC_FUNCTION/1(acc_status) -> Scope4/1, Scope6/5, acc_status/1  "acc_status"
  ACC_FUNCTION/2(acc_torque[NM]) -> acc_torque/1
  ACC_FUNCTION/4(set_speed_out) -> Scope2/1, set_speed_out/1
  ACC_FUNCTION/5(standstill_req) -> standstill_req/1, Scope6/1  "standstill_request"
  IC_VehSpd_HMI/1 -> ACC_FUNCTION/37(IC_VehSpd_HMI)
  ACC_FUNCTION/6(ACC_DriveOff) -> Scope6/2, Scope1/1, ACC_DriveOff/1  "driveoff"
  ACC_FUNCTION/3(acc_brake[ms-2]) -> Scope6/3, Scope3/1, acc_brake/1

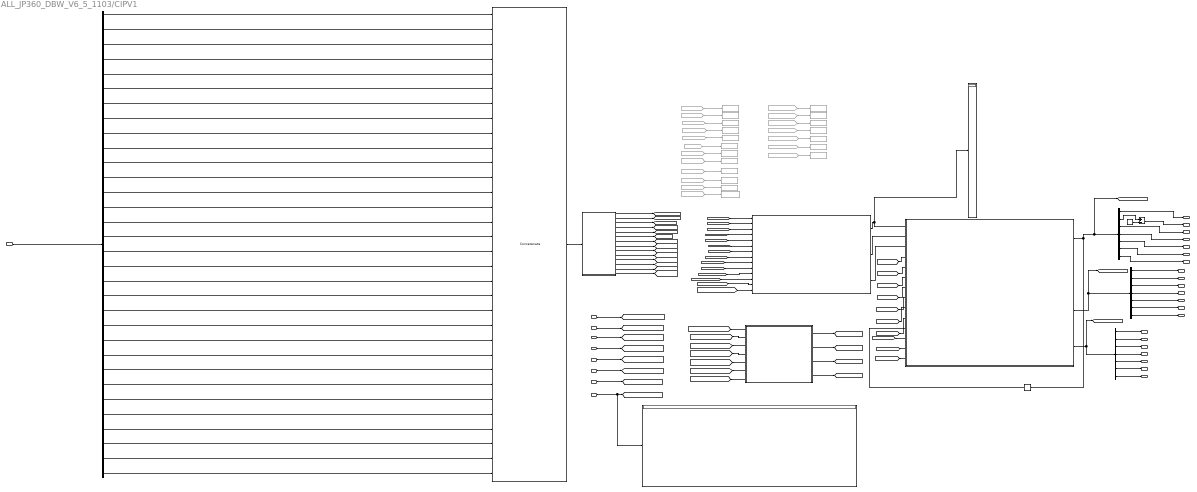
== system ALL_JP360_DBW_V6_5_1103/CIPV1 ==
  note: log
  note: 1、Lane Line Construction：用于提供车道线给后续模块使用，包括感知的车道线和虚拟车道线
      | 输入：ipm_line 、方向盘转角、横摆角速度、车速
      | 输出：左、右、左左、右右车道线。以该格式输出：Y = C0 + C1 * X + 1/2 * C2 * X^2 + 1/6 * C3 * X^3
      | Y为距离参考点的横向距离，X为距离参考点的纵向距离
      | 单位：m
      | C0：近端Y轴坐标，Video_Line_0x_A_dy
      | C1：切线夹角θ，Video_Line_0x_A_ yawangle
      | C2：曲率，Video_Line_0x_ B_hor_curve
      | C3: 曲率变化率，BV_Lin_0x_hor_curvature_alteration
      | 2、filter ：滤掉空目标，概率低的目标，矩形ROI外的目标、相对行驶的目标、不在本车道的静止目标，
      | 并将障碍物分成自车道障碍物，左车道障碍物，右车道障碍物输出
      | 3、Obstacle selection：选取cipv和 相邻障碍物目标，防止CIPV防跳变，替换障碍物类型
  MRR_obj_1_32 : Inport
  Ego_speed : Inport  Port=2
  ESP_YawRate : Inport  Port=3
  IPM_Line_01 : Inport  Port=4
  IPM_Line_02 : Inport  Port=5
  PM_Line_03 : Inport  Port=6
  IPM_Line_04 : Inport  Port=7
  SAS_SteerWheelAngle : Inport  Port=8
  IPM_obj_1_20 : Inport  Port=9
  Add : Sum  Inputs=+-
  Bus Selector : BusSelector  OutputSignals=MRR_ObjID,MRR_ObjDistX,MRR_ObjDistY,MRR_ObjRelVelX,MRR_ObjRelVelY,MRR_ObjType,obj_vaild
  Bus Selector1 : BusSelector  OutputSignals=MRR_ObjID,MRR_ObjDistX,MRR_ObjDistY,MRR_ObjRelVelX,MRR_ObjRelVelY,MRR_ObjType,obj_vaild
  Bus Selector2 : BusSelector  OutputSignals=MRR_ObjID,MRR_ObjDistX,MRR_ObjDistY,MRR_ObjRelVelX,MRR_ObjRelVelY,MRR_ObjType,obj_vaild
  Constant : Constant  Value=4.174  OutDataTypeStr=single
  Delay : Delay  DelayLength=1  InitialCondition=1
  Demux : Demux  Outputs=32
  Display : Display
  Display1 : Display
  From15 : From  Commented=on  GotoTag=MRR_ObjExistProb
  From16 : From  Commented=on  GotoTag=MRR_ObjFusionCamID
  From17 : From  Commented=on  GotoTag=MRR_ObjFusionSig
  From18 : From  Commented=on  GotoTag=MRR_ObjID
  From19 : From  Commented=on  GotoTag=MRR_ObjMovingSts
  From20 : From  Commented=on  GotoTag=MRR_ObjObstacleProb
  From25 : From  Commented=on  GotoTag=MRR_ObjRelAccelX
  From35 : From  Commented=on  GotoTag=MRR_ObjDistX
  From38 : From  Commented=on  GotoTag=MRR_ObjDistY
  From39 : From  Commented=on  GotoTag=MRR_ObjRelAccelY
  From40 : From  Commented=on  GotoTag=MRR_ObjRelVelX
  From41 : From  Commented=on  GotoTag=MRR_ObjRelVelY
  From42 : From  Commented=on  GotoTag=left_line
  From43 : From  Commented=on  GotoTag=right_line
  From44 : From  Commented=on  GotoTag=left_left_line
  From45 : From  Commented=on  GotoTag=right_right_line
  From46 : From  Commented=on  GotoTag=cipv1
  From47 : From  Commented=on  GotoTag=left_obj
  From48 : From  Commented=on  GotoTag=right_obj
  Lane Line Construction1 : Subsystem
  Obstacle selection : Subsystem
  To Workspace : ToWorkspace  Commented=on  VariableName=inputMRR_ObjDistX  SaveFormat=Timeseries  SampleTime=-1
  To Workspace1 : ToWorkspace  Commented=on  VariableName=inputMRR_ObjExistProb  SaveFormat=Timeseries  SampleTime=-1
  To Workspace10 : ToWorkspace  Commented=on  VariableName=inputMRR_ObjRelVelX  SaveFormat=Timeseries  SampleTime=-1
  To Workspace11 : ToWorkspace  Commented=on  VariableName=inputMRR_ObjRelVelY  SaveFormat=Timeseries  SampleTime=-1
  To Workspace12 : ToWorkspace  Commented=on  VariableName=outputLeft_line  SaveFormat=Timeseries  SampleTime=-1
  To Workspace13 : ToWorkspace  Commented=on  VariableName=outputRight_line  SaveFormat=Timeseries  SampleTime=-1
  To Workspace14 : ToWorkspace  Commented=on  VariableName=outputLeft_left_line  SaveFormat=Timeseries  SampleTime=-1
  To Workspace15 : ToWorkspace  Commented=on  VariableName=outputRight_right_line  SaveFormat=Timeseries  SampleTime=-1
  To Workspace16 : ToWorkspace  Commented=on  VariableName=outputCipv1  SaveFormat=Timeseries  SampleTime=-1
  To Workspace17 : ToWorkspace  Commented=on  VariableName=outputLeft_obj  SaveFormat=Timeseries  SampleTime=-1
  To Workspace18 : ToWorkspace  Commented=on  VariableName=outputRight_obj  SaveFormat=Timeseries  SampleTime=-1
  To Workspace2 : ToWorkspace  Commented=on  VariableName=inputMRR_ObjFusionCamID  SaveFormat=Timeseries  SampleTime=-1
  To Workspace3 : ToWorkspace  Commented=on  VariableName=inputMRR_ObjFusionSig  SaveFormat=Timeseries  SampleTime=-1
  To Workspace4 : ToWorkspace  Commented=on  VariableName=inputMRR_ObjID  SaveFormat=Timeseries  SampleTime=-1
  To Workspace5 : ToWorkspace  Commented=on  VariableName=inputMRR_ObjMovingSts  SaveFormat=Timeseries  SampleTime=-1
  To Workspace6 : ToWorkspace  Commented=on  VariableName=inputMRR_ObjObstacleProb  SaveFormat=Timeseries  SampleTime=-1
  To Workspace7 : ToWorkspace  Commented=on  VariableName=inputMRR_ObjDistY  SaveFormat=Timeseries  SampleTime=-1
  To Workspace8 : ToWorkspace  Commented=on  VariableName=inputMRR_ObjRelAccelX  SaveFormat=Timeseries  SampleTime=-1
  To Workspace9 : ToWorkspace  Commented=on  VariableName=inputMRR_ObjRelAccelY  SaveFormat=Timeseries  SampleTime=-1
  Vector Concatenate : Concatenate  NumInputs=32  Mode=Multidimensional array  ConcatenateDimension=2
  filter : Subsystem
  getMrrObjFcn : MATLAB Function  TreatAsAtomicUnit=on
  CIPV_ObjID : Outport
  CIPV_ObjDistX : Outport  Port=2
  CIPV_ObjDistY : Outport  Port=3
  CIPV_ObjRelVelX : Outport  Port=4
  CIPV_ObjRelVelY : Outport  Port=5
  ACC_ObjDetected : Outport  Port=6
  CIPV_ObjType : Outport  Port=7
  Left_closest_ObjID : Outport  Port=8
  Left_closest_ObjDistX : Outport  Port=9
  Left_closest_ObjDistY : Outport  Port=10
  Left_closest_ObjRelVelX : Outport  Port=11
  Left_closest_ObjRelVelY : Outport  Port=12
  ACC_left_ObjDetected : Outport  Port=13
  Left_closest_ObjType : Outport  Port=14
  Right_closest_ObjID : Outport  Port=15
  Right_closest_ObjDistX : Outport  Port=16
  Right_closest_ObjDistY : Outport  Port=17
  Right_closest_ObjRelVelX : Outport  Port=18
  Right_closest_ObjRelVelY : Outport  Port=19
  ACC_right_ObjDetected : Outport  Port=20
  Right_closest_ObjType : Outport  Port=21
  wires:
  MRR_obj_1_32/1 -> Demux/1
  Vector Concatenate/1 -> getMrrObjFcn/1(u)
  Demux/2 -> Vector Concatenate/2
  Demux/1 -> Vector Concatenate/1
  Demux/3 -> Vector Concatenate/3
  Demux/4 -> Vector Concatenate/4
  Demux/5 -> Vector Concatenate/5
  Demux/6 -> Vector Concatenate/6
  Demux/7 -> Vector Concatenate/7
  Demux/8 -> Vector Concatenate/8
  Demux/9 -> Vector Concatenate/9
  Demux/10 -> Vector Concatenate/10
  Demux/11 -> Vector Concatenate/11
  Demux/12 -> Vector Concatenate/12
  Demux/13 -> Vector Concatenate/13
  Demux/14 -> Vector Concatenate/14
  Demux/15 -> Vector Concatenate/15
  Demux/16 -> Vector Concatenate/16
  Demux/17 -> Vector Concatenate/17
  Demux/18 -> Vector Concatenate/18
  Demux/19 -> Vector Concatenate/19
  Demux/20 -> Vector Concatenate/20
  Demux/21 -> Vector Concatenate/21
  Demux/22 -> Vector Concatenate/22
  Demux/23 -> Vector Concatenate/23
  Demux/24 -> Vector Concatenate/24
  Demux/25 -> Vector Concatenate/25
  Demux/26 -> Vector Concatenate/26
  Demux/27 -> Vector Concatenate/27
  Demux/28 -> Vector Concatenate/28
  Demux/29 -> Vector Concatenate/29
  Demux/30 -> Vector Concatenate/30
  Demux/31 -> Vector Concatenate/31
  Demux/32 -> Vector Concatenate/32
  getMrrObjFcn/1(y1) -> [MRR_ObjDistX]
  [MRR_ObjFusionSig] -> filter/5(MRR_ObjFusionSig)  "MRR_ObjFusionSig"
  [MRR_ObjDistY] -> filter/2(MRR_ObjDistY)  "MRR_ObjDistY"
  [MRR_ObjFusionCamID] -> filter/4(MRR_ObjFusionCamID)  "MRR_ObjFusionCamID"
  [MRR_ObjMovingSts] -> filter/6(MRR_ObjMovingSts)
  [MRR_ObjObstacleProb] -> filter/7(MRR_ObjObstacleProb)
  [MRR_ObjRelVelX] -> filter/8(MRR_ObjRelVelX)
  [MRR_ObjRelVelY] -> filter/9(MRR_ObjRelVelY)
  [MRR_ObjType] -> filter/10(MRR_ObjType)
  [MRR_ObjExistProb] -> filter/3(MRR_ObjExistProb)  "MRR_ObjExistProb"
  [MRR_ObjDistX] -> filter/1(MRR_ObjDistX)  "MRR_ObjDistX"
  IPM_Line_01/1 -> [IPM_Line_Left]
  IPM_Line_02/1 -> [IPM_Line_Right]
  PM_Line_03/1 -> [IPM_Line_Left_Left]
  IPM_Line_04/1 -> [IPM_Line_Right_Right]
  SAS_SteerWheelAngle/1 -> [SAS_SteerWheelAngle]
  ESP_YawRate/1 -> [EGO_yaw_rate]
  filter/2(left_lane_obstacles) -> Obstacle selection/2(left_lane_obstacles)
  filter/1(ego_lane_obstacles) -> Display/1, Obstacle selection/1(ego_lane_obstacles)
  filter/3(right_lane_obstacles) -> Obstacle selection/3(right_lane_obstacles)
  Ego_speed/1 -> [Ego_speed]
  [left_line] -> filter/11(left_line)
  [right_line] -> filter/12(right_line)
  [Ego_speed] -> filter/13(Ego_speed)
  getMrrObjFcn/2(y2) -> [MRR_ObjDistY]
  getMrrObjFcn/3(y3) -> [MRR_ObjExistProb]
  getMrrObjFcn/4(y4) -> [MRR_ObjFusionCamID]
  getMrrObjFcn/5(y5) -> [MRR_ObjFusionSig]
  getMrrObjFcn/6(y6) -> [MRR_ObjID]
  getMrrObjFcn/7(y7) -> [MRR_ObjMovingSts]
  getMrrObjFcn/8(y8) -> [MRR_ObjObstacleProb]
  getMrrObjFcn/9(y9) -> [MRR_ObjRelAccelX]
  getMrrObjFcn/10(y10) -> [MRR_ObjRelAccelY]
  getMrrObjFcn/11(y11) -> [MRR_ObjRelVelX]
  getMrrObjFcn/12(y12) -> [MRR_ObjRelVelY]
  getMrrObjFcn/13(y13) -> [MRR_ObjType]
  [MRR_ObjID] -> Obstacle selection/4(MRR_ObjID)
  [MRR_ObjDistX] -> Obstacle selection/5(MRR_ObjDistX)  "MRR_ObjDistX"
  [MRR_ObjDistY] -> Obstacle selection/6(MRR_ObjDistY)  "MRR_ObjDistY"
  [MRR_ObjRelVelX] -> Obstacle selection/7(MRR_ObjRelVelX)
  [MRR_ObjRelVelY] -> Obstacle selection/8(MRR_ObjRelVelY)
  [MRR_ObjType] -> Obstacle selection/9(MRR_ObjType)
  [MRR_ObjUpdFlg] -> Obstacle selection/10(MRR_ObjUpdFlg)
  Obstacle selection/1(cipv1) -> [cipv1], Bus Selector/1, Delay/1
  Delay/1 -> Obstacle selection/11(last_cipv)
  IPM_obj_1_20/1 -> Display1/1, [IPM_obj_1_20]
  getMrrObjFcn/14(y14) -> [MRR_ObjUpdFlg]
  Bus Selector/1 -> CIPV_ObjID/1  "<MRR_ObjID>"
  Add/1 -> CIPV_ObjDistX/1
  Bus Selector/3 -> CIPV_ObjDistY/1  "<MRR_ObjDistY>"
  Bus Selector/4 -> CIPV_ObjRelVelX/1  "<MRR_ObjRelVelX>"
  Bus Selector/5 -> CIPV_ObjRelVelY/1  "<MRR_ObjRelVelY>"
  Bus Selector/6 -> CIPV_ObjType/1  "<MRR_ObjType>"
  Bus Selector/7 -> ACC_ObjDetected/1  "<obj_vaild>"
  Obstacle selection/3(left_obj) -> [left_obj], Bus Selector1/1
  Bus Selector1/1 -> Left_closest_ObjID/1  "<MRR_ObjID>"
  Bus Selector1/2 -> Left_closest_ObjDistX/1  "<MRR_ObjDistX>"
  Bus Selector1/3 -> Left_closest_ObjDistY/1  "<MRR_ObjDistY>"
  Bus Selector1/4 -> Left_closest_ObjRelVelX/1  "<MRR_ObjRelVelX>"
  Bus Selector1/5 -> Left_closest_ObjRelVelY/1  "<MRR_ObjRelVelY>"
  Bus Selector1/7 -> ACC_left_ObjDetected/1  "<obj_vaild>"
  Bus Selector1/6 -> Left_closest_ObjType/1  "<MRR_ObjType>"
  Obstacle selection/4(right_obj) -> [right_obj], Bus Selector2/1
  Bus Selector2/1 -> Right_closest_ObjID/1  "<MRR_ObjID>"
  Bus Selector2/2 -> Right_closest_ObjDistX/1  "<MRR_ObjDistX>"
  Bus Selector2/3 -> Right_closest_ObjDistY/1  "<MRR_ObjDistY>"
  Bus Selector2/4 -> Right_closest_ObjRelVelX/1  "<MRR_ObjRelVelX>"
  Bus Selector2/5 -> Right_closest_ObjRelVelY/1  "<MRR_ObjRelVelY>"
  Bus Selector2/6 -> Right_closest_ObjType/1  "<MRR_ObjType>"
  Bus Selector2/7 -> ACC_right_ObjDetected/1  "<obj_vaild>"
  [IPM_Line_Left] -> Lane Line Construction1/1(IPM_Line_left)
  [SAS_SteerWheelAngle] -> Lane Line Construction1/5(SAS_SteerWheelAngle)
  [Ego_speed] -> Lane Line Construction1/7(EGO_speed)
  Lane Line Construction1/4(right_right_line) -> [right_right_line]
  Lane Line Construction1/3(left_left_line) -> [left_left_line]
  [IPM_Line_Right] -> Lane Line Construction1/2(IPM_Line_right)
  Lane Line Construction1/1(left_line) -> [left_line]  "left_line"
  [IPM_Line_Right_Right] -> Lane Line Construction1/4(IPM_Line_right_right)
  [IPM_Line_Left_Left] -> Lane Line Construction1/3(IPM_Line_left_left)
  Lane Line Construction1/2(right_line) -> [right_line]
  [EGO_yaw_rate] -> Lane Line Construction1/6(EGO_yaw_rate)
  [IPM_obj_1_20] -> filter/14(IPM_objs)
  Constant/1 -> Add/2
  Bus Selector/2 -> Add/1  "<MRR_ObjDistX>"
  From35/1 -> To Workspace/1  "MRR_ObjDistX"
  From38/1 -> To Workspace7/1  "MRR_ObjDistY"
  From15/1 -> To Workspace1/1
  From16/1 -> To Workspace2/1
  From17/1 -> To Workspace3/1
  From18/1 -> To Workspace4/1
  From19/1 -> To Workspace5/1
  From20/1 -> To Workspace6/1
  From25/1 -> To Workspace8/1
  From39/1 -> To Workspace9/1
  From40/1 -> To Workspace10/1
  From41/1 -> To Workspace11/1
  From42/1 -> To Workspace12/1
  From43/1 -> To Workspace13/1
  From44/1 -> To Workspace14/1
  From45/1 -> To Workspace15/1
  From46/1 -> To Workspace16/1
  From47/1 -> To Workspace17/1
  From48/1 -> To Workspace18/1
  [IPM_obj_1_20] -> Obstacle selection/12(IPM_Obj)
  [MRR_ObjFusionSig] -> Obstacle selection/13(MRR_ObjFusionSig)
  [MRR_ObjFusionCamID] -> Obstacle selection/14(MRR_ObjFusionCamID)

== system ALL_JP360_DBW_V6_5_1103/CanbusControl ==
  ACCstatus_in : Inport
  Torque_in : Inport  Port=2
  Brake_in : Inport  Port=3
  LKAstatus_in : Inport  Port=4
  LanelistTorque_in : Inport  Port=5
  AND : Logic  IconShape=distinctive  AllPortsSameDT=off  OutDataTypeStr=boolean
  Add : Sum  Inputs=+-
  Add1 : Sum  Inputs=+-
  Add2 : Sum  Inputs=+-
  Constant{,4..5,8,10,14} (6 alike) : Constant  OutDataTypeStr=boolean
  Constant1 : Constant  Value=4  OutDataTypeStr=int8
  Constant{3,6..7,9,11,13} (6 alike) : Constant  Value=0  OutDataTypeStr=boolean
  Constant12 : Constant  Value=6  OutDataTypeStr=int8
  Constant2 : Constant  Value=3  OutDataTypeStr=int8
  Gain : Gain
  Limit : Subsystem
  OR : Logic  Operator=OR  IconShape=distinctive  AllPortsSameDT=off  OutDataTypeStr=boolean
  Product : Product
  Product1 : Product
  Product2 : Product
  Subsystem4 : Subsystem
  Switch : Switch  SaturateOnIntegerOverflow=off  InputSameDT=off
  Switch{1..5} (5 alike) : Switch  Criteria=u2 ~= 0  SaturateOnIntegerOverflow=off  InputSameDT=off
  Lanelist_Out : Outport
  Torque_Out : Outport  Port=2
  Brake_Out : Outport  Port=3
  Brake_Status : Outport  Port=4
  ACC_StartStop : Outport  Port=5
  Lanelist_Status : Outport  Port=6
  Torque_Status : Outport  Port=7
  wires:
  [status] -> AND/2
  Constant2/1 -> Add/2
  Constant5/1 -> Switch1/3
  Constant6/1 -> Switch/1
  Constant3/1 -> Switch1/1
  Switch/1 -> AND/1
  Product2/1 -> Gain/1
  Torque_in/1 -> Product1/2
  Limit/3(Out3) -> Brake_Out/1, Switch/2
  Product1/1 -> Limit/2(Input1)
  Gain/1 -> Limit/3(Input2)
  Product/1 -> Limit/1(Input)
  AND/1 -> Brake_Status/1
  Brake_in/1 -> Product2/2
  Limit/1(Out1) -> Switch3/2, Lanelist_Out/1
  LanelistTorque_in/1 -> Product/2
  OR/1 -> Product1/1, Product2/1, [status]
  Constant4/1 -> Switch/3
  Add/1 -> Switch1/2
  Subsystem4/1(data1) -> ACC_StartStop/1
  [ACCstatus] -> Subsystem4/1(In1)
  ACCstatus_in/1 -> [ACCstatus]
  [ACCstatus] -> Add/1
  LKAstatus_in/1 -> [LKAstatus]
  [LKAstatus] -> Add1/1
  Add1/1 -> Switch2/2
  Constant7/1 -> Switch2/1
  Constant1/1 -> Add1/2
  Constant8/1 -> Product/1, Switch2/3
  Constant/1 -> Switch3/1
  Constant9/1 -> Switch3/3
  Switch3/1 -> Lanelist_Status/1
  Constant11/1 -> Switch4/3
  Constant10/1 -> Switch4/1
  Limit/2(Out2) -> Switch4/2, Torque_Out/1
  Switch4/1 -> Torque_Status/1
  [ACCstatus] -> Add2/1
  Constant12/1 -> Add2/2
  Add2/1 -> Switch5/2
  Constant13/1 -> Switch5/1
  Constant14/1 -> Switch5/3
  Switch1/1 -> OR/1
  Switch5/1 -> OR/2
